simulink model "SoftManipulatorModel"  (R2019a)
settings: Solver=VariableStepAuto  StartTime=0.0  StopTime=100  FixedStep=0.01  RelTol=1e-3
undefined symbols (not defined in the file): d, dq_init, k, l, m, q_init
libraries: dspinverses x1
(part 1 of 2)
settings Model: Creator=Shaon  LastModifiedBy=Shaon

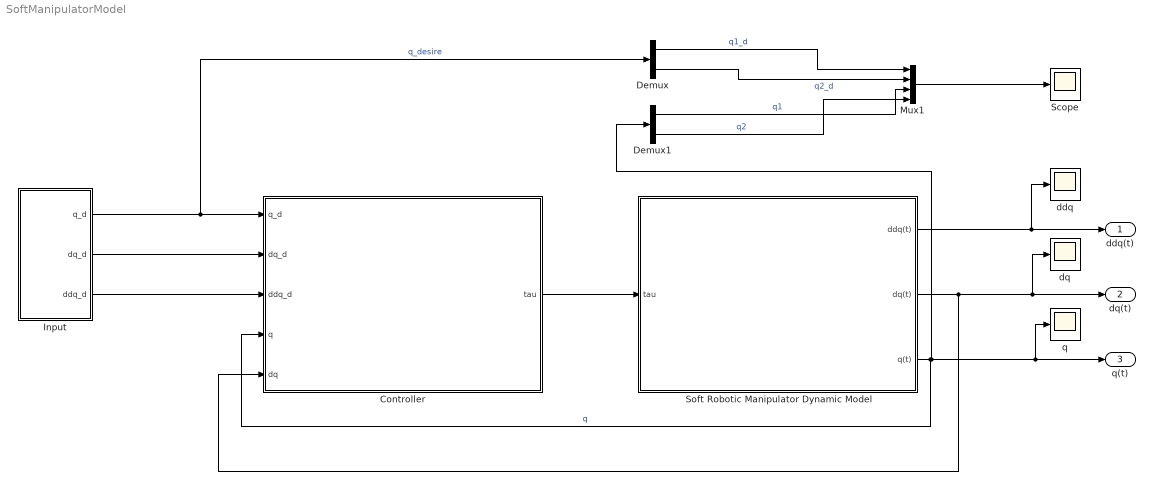
== system SoftManipulatorModel ==
  Controller : Subsystem
  Demux : Demux  Outputs=2
  Demux1 : Demux  Outputs=2
  Input : Subsystem
  Mux1 : Mux
  Scope : Scope
  Soft Robotic Manipulator Dynamic Model : Subsystem
  ddq : Scope
  dq : Scope
  q : Scope
  ddq(t) : Outport
  dq(t) : Outport  Port=2
  q(t) : Outport  Port=3
  wires:
  Soft Robotic Manipulator Dynamic Model/1(ddq(t)) -> ddq/1, ddq(t)/1
  Soft Robotic Manipulator Dynamic Model/2(dq(t)) -> Controller/5(dq), dq/1, dq(t)/1
  Soft Robotic Manipulator Dynamic Model/3(q(t)) -> Demux1/1, q/1, q(t)/1, Controller/4(q)  "q"
  Controller/1(tau) -> Soft Robotic Manipulator Dynamic Model/1(tau)
  Input/1(q_d) -> Demux/1, Controller/1(q_d)  "q_desire"
  Input/2(dq_d) -> Controller/2(dq_d)
  Input/3(ddq_d) -> Controller/3(ddq_d)
  Mux1/1 -> Scope/1
  Demux/1 -> Mux1/1  "q1_d"
  Demux/2 -> Mux1/2  "q2_d"
  Demux1/1 -> Mux1/3  "q1"
  Demux1/2 -> Mux1/4  "q2"

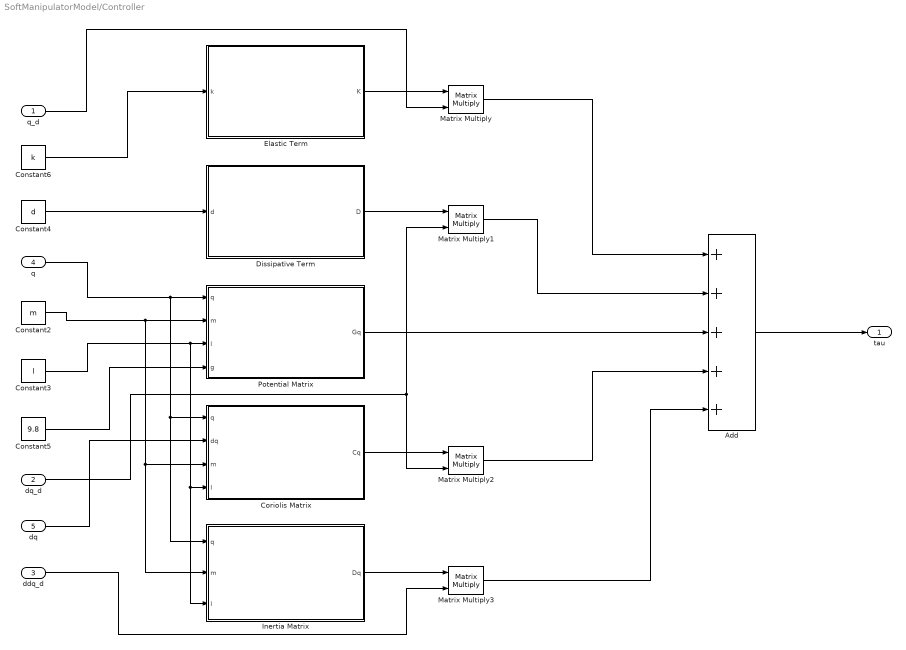
== system SoftManipulatorModel/Controller ==
  q_d : Inport
  dq_d : Inport  Port=2
  ddq_d : Inport  Port=3
  q : Inport  Port=4
  dq : Inport  Port=5
  " Dissipative Term" : MATLAB Function  TreatAsAtomicUnit=on
  Add : Sum  Inputs=+++++
  Constant2 : Constant  Value=m
  Constant3 : Constant  Value=l
  Constant4 : Constant  Value=d
  Constant5 : Constant  Value=9.8
  Constant6 : Constant  Value=k
  Coriolis Matrix : MATLAB Function  TreatAsAtomicUnit=on
  Elastic Term : MATLAB Function  TreatAsAtomicUnit=on
  Inertia Matrix : MATLAB Function  TreatAsAtomicUnit=on
  Matrix Multiply{,1..3} (4 alike) : Product  Multiplication=Matrix(*)
  Potential Matrix : MATLAB Function  TreatAsAtomicUnit=on
  tau : Outport
  wires:
  Elastic Term/1(K) -> Matrix Multiply/1
  " Dissipative Term"/1(D) -> Matrix Multiply1/1
  Potential Matrix/1(Gq) -> Add/3
  Matrix Multiply/1 -> Add/1
  Matrix Multiply1/1 -> Add/2
  Matrix Multiply2/1 -> Add/4
  Matrix Multiply3/1 -> Add/5
  Add/1 -> tau/1
  Coriolis Matrix/1(Cq) -> Matrix Multiply2/1
  Inertia Matrix/1(Dq) -> Matrix Multiply3/1
  Constant6/1 -> Elastic Term/1(k)
  q_d/1 -> Matrix Multiply/2
  Constant4/1 -> " Dissipative Term"/1(d)
  dq_d/1 -> Matrix Multiply1/2, Matrix Multiply2/2
  q/1 -> Inertia Matrix/1(q), Coriolis Matrix/1(q), Potential Matrix/1(q)
  Constant2/1 -> Inertia Matrix/2(m), Coriolis Matrix/3(m), Potential Matrix/2(m)
  Constant3/1 -> Potential Matrix/3(l), Inertia Matrix/3(l), Coriolis Matrix/4(l)
  Constant5/1 -> Potential Matrix/4(g)
  dq/1 -> Coriolis Matrix/2(dq)
  ddq_d/1 -> Matrix Multiply3/2

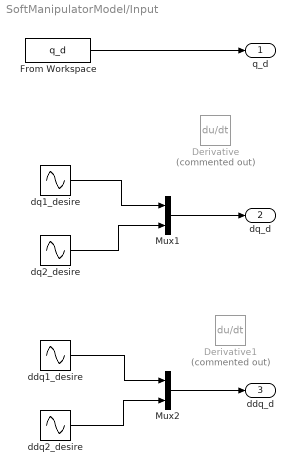
== system SoftManipulatorModel/Input ==
  Derivative : Derivative  Commented=on
  Derivative1 : Derivative  Commented=on
  From Workspace : FromWorkspace  VariableName=q_d  SampleTime=0.1  Interpolate=off  OutputAfterFinalValue=Holding final value
  Mux1 : Mux  Inputs=2
  Mux2 : Mux  Inputs=2
  ddq1_desire : Sin  Amplitude=0  SampleTime=0
  ddq2_desire : Sin  Amplitude=0  SampleTime=0
  dq1_desire : Sin  Amplitude=0  SampleTime=0
  dq2_desire : Sin  Amplitude=0  SampleTime=0
  q_d : Outport
  dq_d : Outport  Port=2
  ddq_d : Outport  Port=3
  wires:
  ddq1_desire/1 -> Mux2/1
  ddq2_desire/1 -> Mux2/2
  Mux2/1 -> ddq_d/1
  Mux1/1 -> dq_d/1
  dq1_desire/1 -> Mux1/1
  dq2_desire/1 -> Mux1/2
  From Workspace/1 -> q_d/1

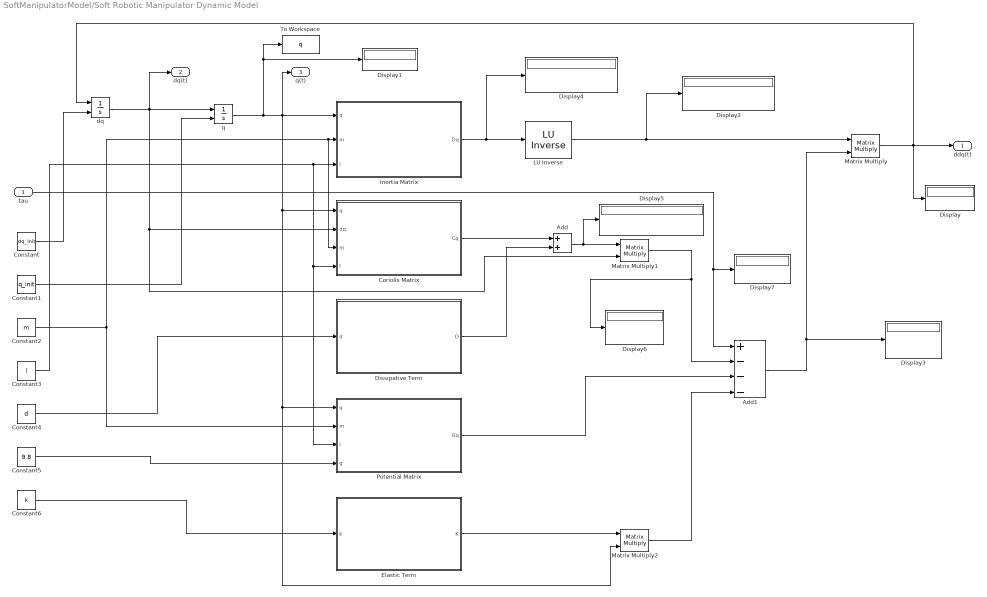
== system SoftManipulatorModel/Soft Robotic Manipulator Dynamic Model ==
  tau : Inport
  " Dissipative Term" : MATLAB Function  TreatAsAtomicUnit=on
  " LU Inverse" : dspinverses/ LU Inverse
      settings: SourceProductName=DSP System Toolbox
  Add : Sum
  Add1 : Sum  Inputs=+---
  Constant : Constant  Value=dq_init
  Constant1 : Constant  Value=q_init
  Constant2 : Constant  Value=m
  Constant3 : Constant  Value=l
  Constant4 : Constant  Value=d
  Constant5 : Constant  Value=9.8
  Constant6 : Constant  Value=k
  Coriolis Matrix : MATLAB Function  TreatAsAtomicUnit=on
  Display{,1..7} (8 alike) : Display
  Elastic Term : MATLAB Function  TreatAsAtomicUnit=on
  Inertia Matrix : MATLAB Function  TreatAsAtomicUnit=on
  Matrix Multiply : Product  Multiplication=Matrix(*)
  Matrix Multiply1 : Product  Multiplication=Matrix(*)
  Matrix Multiply2 : Product  Multiplication=Matrix(*)
  Potential Matrix : MATLAB Function  TreatAsAtomicUnit=on
  To Workspace : ToWorkspace  VariableName=q  SampleTime=-1
      settings: Save2DSignal=2-D array (concatenate along first dimension)
  dq : Integrator  InitialConditionSource=external
  q : Integrator  InitialConditionSource=external
  ddq(t) : Outport
  dq(t) : Outport  Port=2
  q(t) : Outport  Port=3
  wires:
  dq/1 -> dq(t)/1, Coriolis Matrix/2(dq), Matrix Multiply1/2, q/1
  " LU Inverse"/1 -> Display2/1, Matrix Multiply/1
  Coriolis Matrix/1(Cq) -> Add/1
  " Dissipative Term"/1(D) -> Add/2
  Constant5/1 -> Potential Matrix/4(g)
  Constant/1 -> dq/2
  Matrix Multiply1/1 -> Display6/1, Add1/2
  Inertia Matrix/1(Dq) -> Display4/1, " LU Inverse"/1
  tau/1 -> Display7/1, Add1/1
  Potential Matrix/1(Gq) -> Add1/3
  Constant2/1 -> Potential Matrix/2(m), Coriolis Matrix/3(m), Inertia Matrix/2(m)
  Add1/1 -> Matrix Multiply/2, Display3/1
  Constant1/1 -> q/2
  Matrix Multiply/1 -> Display/1, ddq(t)/1, dq/1
  Matrix Multiply2/1 -> Add1/4
  Constant3/1 -> Coriolis Matrix/4(l), Potential Matrix/3(l), Inertia Matrix/3(l)
  Add/1 -> Matrix Multiply1/1, Display5/1
  Constant6/1 -> Elastic Term/1(k)
  Constant4/1 -> " Dissipative Term"/1(d)
  Elastic Term/1(K) -> Matrix Multiply2/1
  q/1 -> Inertia Matrix/1(q), Potential Matrix/1(q), Matrix Multiply2/2, Coriolis Matrix/1(q), q(t)/1, Display1/1, To Workspace/1

== matlab function SoftManipulatorModel/Soft Robotic Manipulator Dynamic Model/Coriolis Matrix ==
  data: q input; Cq output; dq input; m input; l input
function Cq = fcn(q, dq, m, l)

q1 = q(1);
q2 = q(2);
dq1 = dq(1);
dq2 = dq(2);
m1 = m(1);
m2 = m(2);
l1 = l(1);
l2 = l(2);

Cq = zeros(2,2);
% C111 = 0;
% C121 = 0;
% C221 = 0;
% C112 = 0;
% C222 = 0;
% tolerance = 1e-4;
% fake_zero = 1e-3;

% This equation got from Matlab symbolic calculation
% if abs(q1) < tolerance && abs(q2) > tolerance
%     C111 = 0;
%     C121 = -(m2*((l2*sin(conj(q2))*conj(l2)*(cos(q2) - 1))/(4*q2*conj(q2)) - ((l2*cos(q2))/(2*q2) - (l2*sin(q2))/(2*q2^2))*(conj(l1) + (sin(conj(q2))*conj(l2))/(2*conj(q2))) - (l1 + (l2*sin(q2))/(2*q2))*((cos(conj(q2))*conj(l2))/(2*conj(q2)) - (sin(conj(q2))*conj(l2))/(2*conj(q2)^2)) + (l2*conj(l2)*sin(q2)*(cos(conj(q2)) - 1))/(4*q2*conj(q2)) + (l2*conj(l2)*(cos(q2) - 1)*(cos(conj(q2)) - 1))/(4*q2*conj(q2)^2) + (l2*conj(l2)*(cos(q2) - 1)*(cos(conj(q2)) - 1))/(4*q2^2*conj(q2))))/2;
%     C221 = -m2*((l2*sin(q2)*(conj(l1) + (sin(conj(q2))*conj(l2))/(2*conj(q2))))/(2*q2^2) - (l2*cos(q2)*(conj(l1) + (sin(conj(q2))*conj(l2))/(2*conj(q2))))/(2*q2) - (l2*sin(q2)*((cos(conj(q2))*conj(l2))/(2*conj(q2)) - (sin(conj(q2))*conj(l2))/(2*conj(q2)^2)))/(2*q2) + (l2*sin(conj(q2))*conj(l2)*(cos(q2) - 1))/(4*q2*conj(q2)) + (l2*conj(l2)*sin(q2)*(cos(conj(q2)) - 1))/(4*q2*conj(q2)) + (l2*conj(l2)*(cos(q2) - 1)*(cos(conj(q2)) - 1))/(4*q2*conj(q2)^2) + (l2*conj(l2)*(cos(q2) - 1)*(cos(conj(q2)) - 1))/(4*q2^2*conj(q2)));
%     C112 = (m2*((l2*sin(conj(q2))*conj(l2)*(cos(q2) - 1))/(4*q2*conj(q2)) - ((l2*cos(q2))/(2*q2) - (l2*sin(q2))/(2*q2^2))*(conj(l1) + (sin(conj(q2))*conj(l2))/(2*conj(q2))) - (l1 + (l2*sin(q2))/(2*q2))*((cos(conj(q2))*conj(l2))/(2*conj(q2)) - (sin(conj(q2))*conj(l2))/(2*conj(q2)^2)) + (l2*conj(l2)*sin(q2)*(cos(conj(q2)) - 1))/(4*q2*conj(q2)) + (l2*conj(l2)*(cos(q2) - 1)*(cos(conj(q2)) - 1))/(4*q2*conj(q2)^2) + (l2*conj(l2)*(cos(q2) - 1)*(cos(conj(q2)) - 1))/(4*q2^2*conj(q2))))/2;
%     C222 = -(m2*((l2*sin(conj(q2))*conj(l2)*(cos(q2) - 1))/(4*q2*conj(q2)) + (l2*conj(l2)*sin(q2)*(cos(conj(q2)) - 1))/(4*q2*conj(q2)) + (l2*conj(l2)*(cos(q2) - 1)*(cos(conj(q2)) - 1))/(4*q2*conj(q2)^2) + (l2*conj(l2)*(cos(q2) - 1)*(cos(conj(q2)) - 1))/(4*q2^2*conj(q2)) - (l2*cos(conj(q2))*conj(l2)*sin(q2))/(4*q2*conj(q2)) - (l2*sin(conj(q2))*conj(l2)*cos(q2))/(4*q2*conj(q2)) + (l2*sin(conj(q2))*conj(l2)*sin(q2))/(4*q2*conj(q2)^2) + (l2*sin(conj(q2))*conj(l2)*sin(q2))/(4*q2^2*conj(q2))))/2;
% elseif abs(q1) < tolerance && abs(q2) < tolerance
%     C111 = 0;
%     C121 = 0;
%     C221 = 0;
%     C112 = 0;
%     C222 = 0;
% elseif abs(q1) > tolerance && abs(q2) < tolerance
%     C111 = m2*(((sin(conj(q1))*conj(l2))/2 - (conj(l1)*(cos(conj(q1)) - 1))/conj(q1))*((l2*cos(q1))/2 + (l1*sin(q1))/q1 + (l1*(cos(q1) - 1))/q1^2) + ((l2*sin(q1))/2 - (l1*(cos(q1) - 1))/q1)*((cos(conj(q1))*conj(l2))/2 + (sin(conj(q1))*conj(l1))/conj(q1) + (conj(l1)*(cos(conj(q1)) - 1))/conj(q1)^2) - ((cos(conj(q1))*conj(l2))/2 + (sin(conj(q1))*conj(l1))/conj(q1))*((l2*sin(q1))/2 - (l1*cos(q1))/q1 + (l1*sin(q1))/q1^2) - ((l2*cos(q1))/2 + (l1*sin(q1))/q1)*((sin(conj(q1))*conj(l2))/2 - (cos(conj(q1))*conj(l1))/conj(q1) + (sin(conj(q1))*conj(l1))/conj(q1)^2)) - m1*((l1*sin(conj(q1))*conj(l1)*(cos(q1) - 1))/(4*q1*conj(q1)) + (l1*conj(l1)*sin(q1)*(cos(conj(q1)) - 1))/(4*q1*conj(q1)) + (l1*conj(l1)*(cos(q1) - 1)*(cos(conj(q1)) - 1))/(4*q1*conj(q1)^2) + (l1*conj(l1)*(cos(q1) - 1)*(cos(conj(q1)) - 1))/(4*q1^2*conj(q1)) - (l1*cos(conj(q1))*conj(l1)*sin(q1))/(4*q1*conj(q1)) - (l1*sin(conj(q1))*conj(l1)*cos(q1))/(4*q1*conj(q1)) + (l1*sin(conj(q1))*conj(l1)*sin(q1))/(4*q1*conj(q1)^2) + (l1*sin(conj(q1))*conj(l1)*sin(q1))/(4*q1^2*conj(q1)));
%     C121 = 0;
%     C221 = 0;
%     C112 = m2*((cos(conj(q1))*conj(l2)*((l2*sin(q1))/2 - (l1*(cos(q1) - 1))/q1))/2 - (cos(conj(q1))*conj(l2)*((l2*sin(q1))/2 - (l1*cos(q1))/q1 + (l1*sin(q1))/q1^2))/2 + (sin(conj(q1))*conj(l2)*((l2*cos(q1))/2 + (l1*sin(q1))/q1 + (l1*(cos(q1) - 1))/q1^2))/2 - (sin(conj(q1))*conj(l2)*((l2*cos(q1))/2 + (l1*sin(q1))/q1))/2);
%     C222 = 0;
% elseif abs(q1) > tolerance && abs(q2) > tolerance
%     C111 = m2*(((l1*sin(q1))/q1 + (l2*cos(q1)*sin(q2))/(2*q2) + (l2*sin(q1)*(cos(q2) - 1))/(2*q2))*((cos(conj(q1))*conj(l1))/conj(q1) - (sin(conj(q1))*conj(l1))/conj(q1)^2 + (cos(conj(q1))*conj(l2)*(cos(conj(q2)) - 1))/(2*conj(q2)) - (sin(conj(q1))*sin(conj(q2))*conj(l2))/(2*conj(q2))) - ((conj(l1)*(cos(conj(q1)) - 1))/conj(q1) + (cos(conj(q1))*conj(l2)*(cos(conj(q2)) - 1))/(2*conj(q2)) - (sin(conj(q1))*sin(conj(q2))*conj(l2))/(2*conj(q2)))*((l1*sin(q1))/q1 + (l1*(cos(q1) - 1))/q1^2 + (l2*cos(q1)*sin(q2))/(2*q2) + (l2*sin(q1)*(cos(q2) - 1))/(2*q2)) - ((l1*(cos(q1) - 1))/q1 - (l2*sin(q1)*sin(q2))/(2*q2) + (l2*cos(q1)*(cos(q2) - 1))/(2*q2))*((sin(conj(q1))*conj(l1))/conj(q1) + (conj(l1)*(cos(conj(q1)) - 1))/conj(q1)^2 + (sin(conj(q1))*conj(l2)*(cos(conj(q2)) - 1))/(2*conj(q2)) + (cos(conj(q1))*sin(conj(q2))*conj(l2))/(2*conj(q2))) + ((sin(conj(q1))*conj(l1))/conj(q1) + (sin(conj(q1))*conj(l2)*(cos(conj(q2)) - 1))/(2*conj(q2)) + (cos(conj(q1))*sin(conj(q2))*conj(l2))/(2*conj(q2)))*((l1*cos(q1))/q1 - (l1*sin(q1))/q1^2 - (l2*sin(q1)*sin(q2))/(2*q2) + (l2*cos(q1)*(cos(q2) - 1))/(2*q2))) - m1*((l1*sin(conj(q1))*conj(l1)*(cos(q1) - 1))/(4*q1*conj(q1)) + (l1*conj(l1)*sin(q1)*(cos(conj(q1)) - 1))/(4*q1*conj(q1)) + (l1*conj(l1)*(cos(q1) - 1)*(cos(conj(q1)) - 1))/(4*q1*conj(q1)^2) + (l1*conj(l1)*(cos(q1) - 1)*(cos(conj(q1)) - 1))/(4*q1^2*conj(q1)) - (l1*cos(conj(q1))*conj(l1)*sin(q1))/(4*q1*conj(q1)) - (l1*sin(conj(q1))*conj(l1)*cos(q1))/(4*q1*conj(q1)) + (l1*sin(conj(q1))*conj(l1)*sin(q1))/(4*q1*conj(q1)^2) + (l1*sin(conj(q1))*conj(l1)*sin(q1))/(4*q1^2*conj(q1)));
%     C121 = -(m2*(((l1*sin(q1))/q1 + (l2*cos(q1)*sin(q2))/(2*q2) + (l2*sin(q1)*(cos(q2) - 1))/(2*q2))*((sin(conj(q1))*conj(l2)*(cos(conj(q2)) - 1))/(2*conj(q2)^2) - (cos(conj(q1))*cos(conj(q2))*conj(l2))/(2*conj(q2)) + (cos(conj(q1))*sin(conj(q2))*conj(l2))/(2*conj(q2)^2) + (sin(conj(q1))*sin(conj(q2))*conj(l2))/(2*conj(q2))) + ((sin(conj(q1))*conj(l1))/conj(q1) + (sin(conj(q1))*conj(l2)*(cos(conj(q2)) - 1))/(2*conj(q2)) + (cos(conj(q1))*sin(conj(q2))*conj(l2))/(2*conj(q2)))*((l2*cos(q1)*sin(q2))/(2*q2^2) - (l2*cos(q1)*cos(q2))/(2*q2) + (l2*sin(q1)*sin(q2))/(2*q2) + (l2*sin(q1)*(cos(q2) - 1))/(2*q2^2)) + ((l1*(cos(q1) - 1))/q1 - (l2*sin(q1)*sin(q2))/(2*q2) + (l2*cos(q1)*(cos(q2) - 1))/(2*q2))*((cos(conj(q1))*conj(l2)*(cos(conj(q2)) - 1))/(2*conj(q2)^2) + (cos(conj(q1))*sin(conj(q2))*conj(l2))/(2*conj(q2)) + (cos(conj(q2))*sin(conj(q1))*conj(l2))/(2*conj(q2)) - (sin(conj(q1))*sin(conj(q2))*conj(l2))/(2*conj(q2)^2)) + ((conj(l1)*(cos(conj(q1)) - 1))/conj(q1) + (cos(conj(q1))*conj(l2)*(cos(conj(q2)) - 1))/(2*conj(q2)) - (sin(conj(q1))*sin(conj(q2))*conj(l2))/(2*conj(q2)))*((l2*cos(q1)*sin(q2))/(2*q2) + (l2*cos(q2)*sin(q1))/(2*q2) - (l2*sin(q1)*sin(q2))/(2*q2^2) + (l2*cos(q1)*(cos(q2) - 1))/(2*q2^2))))/2;
%     C221 = -m2*(((l2*cos(q1)*sin(q2))/(2*q2) + (l2*sin(q1)*(cos(q2) - 1))/(2*q2))*((sin(conj(q1))*conj(l2)*(cos(conj(q2)) - 1))/(2*conj(q2)^2) - (cos(conj(q1))*cos(conj(q2))*conj(l2))/(2*conj(q2)) + (cos(conj(q1))*sin(conj(q2))*conj(l2))/(2*conj(q2)^2) + (sin(conj(q1))*sin(conj(q2))*conj(l2))/(2*conj(q2))) - ((l2*sin(q1)*sin(q2))/(2*q2) - (l2*cos(q1)*(cos(q2) - 1))/(2*q2))*((cos(conj(q1))*conj(l2)*(cos(conj(q2)) - 1))/(2*conj(q2)^2) + (cos(conj(q1))*sin(conj(q2))*conj(l2))/(2*conj(q2)) + (cos(conj(q2))*sin(conj(q1))*conj(l2))/(2*conj(q2)) - (sin(conj(q1))*sin(conj(q2))*conj(l2))/(2*conj(q2)^2)) + ((sin(conj(q1))*conj(l1))/conj(q1) + (sin(conj(q1))*conj(l2)*(cos(conj(q2)) - 1))/(2*conj(q2)) + (cos(conj(q1))*sin(conj(q2))*conj(l2))/(2*conj(q2)))*((l2*cos(q1)*sin(q2))/(2*q2^2) - (l2*cos(q1)*cos(q2))/(2*q2) + (l2*sin(q1)*sin(q2))/(2*q2) + (l2*sin(q1)*(cos(q2) - 1))/(2*q2^2)) + ((conj(l1)*(cos(conj(q1)) - 1))/conj(q1) + (cos(conj(q1))*conj(l2)*(cos(conj(q2)) - 1))/(2*conj(q2)) - (sin(conj(q1))*sin(conj(q2))*conj(l2))/(2*conj(q2)))*((l2*cos(q1)*sin(q2))/(2*q2) + (l2*cos(q2)*sin(q1))/(2*q2) - (l2*sin(q1)*sin(q2))/(2*q2^2) + (l2*cos(q1)*(cos(q2) - 1))/(2*q2^2)));
%     C112 = (m2*(((l1*sin(q1))/q1 + (l2*cos(q1)*sin(q2))/(2*q2) + (l2*sin(q1)*(cos(q2) - 1))/(2*q2))*((sin(conj(q1))*conj(l2)*(cos(conj(q2)) - 1))/(2*conj(q2)^2) - (cos(conj(q1))*cos(conj(q2))*conj(l2))/(2*conj(q2)) + (cos(conj(q1))*sin(conj(q2))*conj(l2))/(2*conj(q2)^2) + (sin(conj(q1))*sin(conj(q2))*conj(l2))/(2*conj(q2))) + ((sin(conj(q1))*conj(l1))/conj(q1) + (sin(conj(q1))*conj(l2)*(cos(conj(q2)) - 1))/(2*conj(q2)) + (cos(conj(q1))*sin(conj(q2))*conj(l2))/(2*conj(q2)))*((l2*cos(q1)*sin(q2))/(2*q2^2) - (l2*cos(q1)*cos(q2))/(2*q2) + (l2*sin(q1)*sin(q2))/(2*q2) + (l2*sin(q1)*(cos(q2) - 1))/(2*q2^2)) + ((l1*(cos(q1) - 1))/q1 - (l2*sin(q1)*sin(q2))/(2*q2) + (l2*cos(q1)*(cos(q2) - 1))/(2*q2))*((cos(conj(q1))*conj(l2)*(cos(conj(q2)) - 1))/(2*conj(q2)^2) + (cos(conj(q1))*sin(conj(q2))*conj(l2))/(2*conj(q2)) + (cos(conj(q2))*sin(conj(q1))*conj(l2))/(2*conj(q2)) - (sin(conj(q1))*sin(conj(q2))*conj(l2))/(2*conj(q2)^2)) + ((conj(l1)*(cos(conj(q1)) - 1))/conj(q1) + (cos(conj(q1))*conj(l2)*(cos(conj(q2)) - 1))/(2*conj(q2)) - (sin(conj(q1))*sin(conj(q2))*conj(l2))/(2*conj(q2)))*((l2*cos(q1)*sin(q2))/(2*q2) + (l2*cos(q2)*sin(q1))/(2*q2) - (l2*sin(q1)*sin(q2))/(2*q2^2) + (l2*cos(q1)*(cos(q2) - 1))/(2*q2^2))))/2 - m2*(((sin(conj(q1))*conj(l2)*(cos(conj(q2)) - 1))/(2*conj(q2)) + (cos(conj(q1))*sin(conj(q2))*conj(l2))/(2*conj(q2)))*((l1*(cos(q1) - 1))/q1 - (l2*sin(q1)*sin(q2))/(2*q2) + (l2*cos(q1)*(cos(q2) - 1))/(2*q2)) - ((sin(conj(q1))*conj(l2)*(cos(conj(q2)) - 1))/(2*conj(q2)) + (cos(conj(q1))*sin(conj(q2))*conj(l2))/(2*conj(q2)))*((l1*cos(q1))/q1 - (l1*sin(q1))/q1^2 - (l2*sin(q1)*sin(q2))/(2*q2) + (l2*cos(q1)*(cos(q2) - 1))/(2*q2)) + ((cos(conj(q1))*conj(l2)*(cos(conj(q2)) - 1))/(2*conj(q2)) - (sin(conj(q1))*sin(conj(q2))*conj(l2))/(2*conj(q2)))*((l1*sin(q1))/q1 + (l1*(cos(q1) - 1))/q1^2 + (l2*cos(q1)*sin(q2))/(2*q2) + (l2*sin(q1)*(cos(q2) - 1))/(2*q2)) - ((cos(conj(q1))*conj(l2)*(cos(conj(q2)) - 1))/(2*conj(q2)) - (sin(conj(q1))*sin(conj(q2))*conj(l2))/(2*conj(q2)))*((l1*sin(q1))/q1 + (l2*cos(q1)*sin(q2))/(2*q2) + (l2*sin(q1)*(cos(q2) - 1))/(2*q2)));
%     C222 = -(m2*(((l2*cos(q1)*sin(q2))/(2*q2) + (l2*sin(q1)*(cos(q2) - 1))/(2*q2))*((sin(conj(q1))*conj(l2)*(cos(conj(q2)) - 1))/(2*conj(q2)^2) - (cos(conj(q1))*cos(conj(q2))*conj(l2))/(2*conj(q2)) + (cos(conj(q1))*sin(conj(q2))*conj(l2))/(2*conj(q2)^2) + (sin(conj(q1))*sin(conj(q2))*conj(l2))/(2*conj(q2))) - ((l2*sin(q1)*sin(q2))/(2*q2) - (l2*cos(q1)*(cos(q2) - 1))/(2*q2))*((cos(conj(q1))*conj(l2)*(cos(conj(q2)) - 1))/(2*conj(q2)^2) + (cos(conj(q1))*sin(conj(q2))*conj(l2))/(2*conj(q2)) + (cos(conj(q2))*sin(conj(q1))*conj(l2))/(2*conj(q2)) - (sin(conj(q1))*sin(conj(q2))*conj(l2))/(2*conj(q2)^2)) + ((cos(conj(q1))*conj(l2)*(cos(conj(q2)) - 1))/(2*conj(q2)) - (sin(conj(q1))*sin(conj(q2))*conj(l2))/(2*conj(q2)))*((l2*cos(q1)*sin(q2))/(2*q2) + (l2*cos(q2)*sin(q1))/(2*q2) - (l2*sin(q1)*sin(q2))/(2*q2^2) + (l2*cos(q1)*(cos(q2) - 1))/(2*q2^2)) + ((sin(conj(q1))*conj(l2)*(cos(conj(q2)) - 1))/(2*conj(q2)) + (cos(conj(q1))*sin(conj(q2))*conj(l2))/(2*conj(q2)))*((l2*cos(q1)*sin(q2))/(2*q2^2) - (l2*cos(q1)*cos(q2))/(2*q2) + (l2*sin(q1)*sin(q2))/(2*q2) + (l2*sin(q1)*(cos(q2) - 1))/(2*q2^2))))/2;
% end

% if abs(q1) < tolerance && abs(q2) > tolerance
%     if q1 < 0
%         q1 = -fake_zero;
%     else
%         q1 = fake_zero;
%     end
% elseif abs(q1) < tolerance && abs(q2) < tolerance
%     if q1 < 0
%         q1 = -fake_zero;
%     else
%         q1 = fake_zero;
%     end
%     
%     if q2 < 0
%         q2 = -fake_zero;
%     else
%         q2 = fake_zero;
%     end
% elseif abs(q1) > tolerance && abs(q2) < tolerance
%     if q2 < 0
%         q2 = -fake_zero;
%     else
%         q2 = fake_zero;
%     end
% end

C111 = m2*(((l1*sin(q1))/q1 + (l2*cos(q1)*sin(q2))/(2*q2) + (l2*sin(q1)*(cos(q2) - 1))/(2*q2))*((cos(conj(q1))*conj(l1))/conj(q1) - (sin(conj(q1))*conj(l1))/conj(q1)^2 + (cos(conj(q1))*conj(l2)*(cos(conj(q2)) - 1))/(2*conj(q2)) - (sin(conj(q1))*sin(conj(q2))*conj(l2))/(2*conj(q2))) - ((conj(l1)*(cos(conj(q1)) - 1))/conj(q1) + (cos(conj(q1))*conj(l2)*(cos(conj(q2)) - 1))/(2*conj(q2)) - (sin(conj(q1))*sin(conj(q2))*conj(l2))/(2*conj(q2)))*((l1*sin(q1))/q1 + (l1*(cos(q1) - 1))/q1^2 + (l2*cos(q1)*sin(q2))/(2*q2) + (l2*sin(q1)*(cos(q2) - 1))/(2*q2)) - ((l1*(cos(q1) - 1))/q1 - (l2*sin(q1)*sin(q2))/(2*q2) + (l2*cos(q1)*(cos(q2) - 1))/(2*q2))*((sin(conj(q1))*conj(l1))/conj(q1) + (conj(l1)*(cos(conj(q1)) - 1))/conj(q1)^2 + (sin(conj(q1))*conj(l2)*(cos(conj(q2)) - 1))/(2*conj(q2)) + (cos(conj(q1))*sin(conj(q2))*conj(l2))/(2*conj(q2))) + ((sin(conj(q1))*conj(l1))/conj(q1) + (sin(conj(q1))*conj(l2)*(cos(conj(q2)) - 1))/(2*conj(q2)) + (cos(conj(q1))*sin(conj(q2))*conj(l2))/(2*conj(q2)))*((l1*cos(q1))/q1 - (l1*sin(q1))/q1^2 - (l2*sin(q1)*sin(q2))/(2*q2) + (l2*cos(q1)*(cos(q2) - 1))/(2*q2))) - m1*((l1*sin(conj(q1))*conj(l1)*(cos(q1) - 1))/(4*q1*conj(q1)) + (l1*conj(l1)*sin(q1)*(cos(conj(q1)) - 1))/(4*q1*conj(q1)) + (l1*conj(l1)*(cos(q1) - 1)*(cos(conj(q1)) - 1))/(4*q1*conj(q1)^2) + (l1*conj(l1)*(cos(q1) - 1)*(cos(conj(q1)) - 1))/(4*q1^2*conj(q1)) - (l1*cos(conj(q1))*conj(l1)*sin(q1))/(4*q1*conj(q1)) - (l1*sin(conj(q1))*conj(l1)*cos(q1))/(4*q1*conj(q1)) + (l1*sin(conj(q1))*conj(l1)*sin(q1))/(4*q1*conj(q1)^2) + (l1*sin(conj(q1))*conj(l1)*sin(q1))/(4*q1^2*conj(q1)));
C121 = -(m2*(((l1*sin(q1))/q1 + (l2*cos(q1)*sin(q2))/(2*q2) + (l2*sin(q1)*(cos(q2) - 1))/(2*q2))*((sin(conj(q1))*conj(l2)*(cos(conj(q2)) - 1))/(2*conj(q2)^2) - (cos(conj(q1))*cos(conj(q2))*conj(l2))/(2*conj(q2)) + (cos(conj(q1))*sin(conj(q2))*conj(l2))/(2*conj(q2)^2) + (sin(conj(q1))*sin(conj(q2))*conj(l2))/(2*conj(q2))) + ((sin(conj(q1))*conj(l1))/conj(q1) + (sin(conj(q1))*conj(l2)*(cos(conj(q2)) - 1))/(2*conj(q2)) + (cos(conj(q1))*sin(conj(q2))*conj(l2))/(2*conj(q2)))*((l2*cos(q1)*sin(q2))/(2*q2^2) - (l2*cos(q1)*cos(q2))/(2*q2) + (l2*sin(q1)*sin(q2))/(2*q2) + (l2*sin(q1)*(cos(q2) - 1))/(2*q2^2)) + ((l1*(cos(q1) - 1))/q1 - (l2*sin(q1)*sin(q2))/(2*q2) + (l2*cos(q1)*(cos(q2) - 1))/(2*q2))*((cos(conj(q1))*conj(l2)*(cos(conj(q2)) - 1))/(2*conj(q2)^2) + (cos(conj(q1))*sin(conj(q2))*conj(l2))/(2*conj(q2)) + (cos(conj(q2))*sin(conj(q1))*conj(l2))/(2*conj(q2)) - (sin(conj(q1))*sin(conj(q2))*conj(l2))/(2*conj(q2)^2)) + ((conj(l1)*(cos(conj(q1)) - 1))/conj(q1) + (cos(conj(q1))*conj(l2)*(cos(conj(q2)) - 1))/(2*conj(q2)) - (sin(conj(q1))*sin(conj(q2))*conj(l2))/(2*conj(q2)))*((l2*cos(q1)*sin(q2))/(2*q2) + (l2*cos(q2)*sin(q1))/(2*q2) - (l2*sin(q1)*sin(q2))/(2*q2^2) + (l2*cos(q1)*(cos(q2) - 1))/(2*q2^2))))/2;
C221 = -m2*(((l2*cos(q1)*sin(q2))/(2*q2) + (l2*sin(q1)*(cos(q2) - 1))/(2*q2))*((sin(conj(q1))*conj(l2)*(cos(conj(q2)) - 1))/(2*conj(q2)^2) - (cos(conj(q1))*cos(conj(q2))*conj(l2))/(2*conj(q2)) + (cos(conj(q1))*sin(conj(q2))*conj(l2))/(2*conj(q2)^2) + (sin(conj(q1))*sin(conj(q2))*conj(l2))/(2*conj(q2))) - ((l2*sin(q1)*sin(q2))/(2*q2) - (l2*cos(q1)*(cos(q2) - 1))/(2*q2))*((cos(conj(q1))*conj(l2)*(cos(conj(q2)) - 1))/(2*conj(q2)^2) + (cos(conj(q1))*sin(conj(q2))*conj(l2))/(2*conj(q2)) + (cos(conj(q2))*sin(conj(q1))*conj(l2))/(2*conj(q2)) - (sin(conj(q1))*sin(conj(q2))*conj(l2))/(2*conj(q2)^2)) + ((sin(conj(q1))*conj(l1))/conj(q1) + (sin(conj(q1))*conj(l2)*(cos(conj(q2)) - 1))/(2*conj(q2)) + (cos(conj(q1))*sin(conj(q2))*conj(l2))/(2*conj(q2)))*((l2*cos(q1)*sin(q2))/(2*q2^2) - (l2*cos(q1)*cos(q2))/(2*q2) + (l2*sin(q1)*sin(q2))/(2*q2) + (l2*sin(q1)*(cos(q2) - 1))/(2*q2^2)) + ((conj(l1)*(cos(conj(q1)) - 1))/conj(q1) + (cos(conj(q1))*conj(l2)*(cos(conj(q2)) - 1))/(2*conj(q2)) - (sin(conj(q1))*sin(conj(q2))*conj(l2))/(2*conj(q2)))*((l2*cos(q1)*sin(q2))/(2*q2) + (l2*cos(q2)*sin(q1))/(2*q2) - (l2*sin(q1)*sin(q2))/(2*q2^2) + (l2*cos(q1)*(cos(q2) - 1))/(2*q2^2)));
C112 = (m2*(((l1*sin(q1))/q1 + (l2*cos(q1)*sin(q2))/(2*q2) + (l2*sin(q1)*(cos(q2) - 1))/(2*q2))*((sin(conj(q1))*conj(l2)*(cos(conj(q2)) - 1))/(2*conj(q2)^2) - (cos(conj(q1))*cos(conj(q2))*conj(l2))/(2*conj(q2)) + (cos(conj(q1))*sin(conj(q2))*conj(l2))/(2*conj(q2)^2) + (sin(conj(q1))*sin(conj(q2))*conj(l2))/(2*conj(q2))) + ((sin(conj(q1))*conj(l1))/conj(q1) + (sin(conj(q1))*conj(l2)*(cos(conj(q2)) - 1))/(2*conj(q2)) + (cos(conj(q1))*sin(conj(q2))*conj(l2))/(2*conj(q2)))*((l2*cos(q1)*sin(q2))/(2*q2^2) - (l2*cos(q1)*cos(q2))/(2*q2) + (l2*sin(q1)*sin(q2))/(2*q2) + (l2*sin(q1)*(cos(q2) - 1))/(2*q2^2)) + ((l1*(cos(q1) - 1))/q1 - (l2*sin(q1)*sin(q2))/(2*q2) + (l2*cos(q1)*(cos(q2) - 1))/(2*q2))*((cos(conj(q1))*conj(l2)*(cos(conj(q2)) - 1))/(2*conj(q2)^2) + (cos(conj(q1))*sin(conj(q2))*conj(l2))/(2*conj(q2)) + (cos(conj(q2))*sin(conj(q1))*conj(l2))/(2*conj(q2)) - (sin(conj(q1))*sin(conj(q2))*conj(l2))/(2*conj(q2)^2)) + ((conj(l1)*(cos(conj(q1)) - 1))/conj(q1) + (cos(conj(q1))*conj(l2)*(cos(conj(q2)) - 1))/(2*conj(q2)) - (sin(conj(q1))*sin(conj(q2))*conj(l2))/(2*conj(q2)))*((l2*cos(q1)*sin(q2))/(2*q2) + (l2*cos(q2)*sin(q1))/(2*q2) - (l2*sin(q1)*sin(q2))/(2*q2^2) + (l2*cos(q1)*(cos(q2) - 1))/(2*q2^2))))/2 - m2*(((sin(conj(q1))*conj(l2)*(cos(conj(q2)) - 1))/(2*conj(q2)) + (cos(conj(q1))*sin(conj(q2))*conj(l2))/(2*conj(q2)))*((l1*(cos(q1) - 1))/q1 - (l2*sin(q1)*sin(q2))/(2*q2) + (l2*cos(q1)*(cos(q2) - 1))/(2*q2)) - ((sin(conj(q1))*conj(l2)*(cos(conj(q2)) - 1))/(2*conj(q2)) + (cos(conj(q1))*sin(conj(q2))*conj(l2))/(2*conj(q2)))*((l1*cos(q1))/q1 - (l1*sin(q1))/q1^2 - (l2*sin(q1)*sin(q2))/(2*q2) + (l2*cos(q1)*(cos(q2) - 1))/(2*q2)) + ((cos(conj(q1))*conj(l2)*(cos(conj(q2)) - 1))/(2*conj(q2)) - (sin(conj(q1))*sin(conj(q2))*conj(l2))/(2*conj(q2)))*((l1*sin(q1))/q1 + (l1*(cos(q1) - 1))/q1^2 + (l2*cos(q1)*sin(q2))/(2*q2) + (l2*sin(q1)*(cos(q2) - 1))/(2*q2)) - ((cos(conj(q1))*conj(l2)*(cos(conj(q2)) - 1))/(2*conj(q2)) - (sin(conj(q1))*sin(conj(q2))*conj(l2))/(2*conj(q2)))*((l1*sin(q1))/q1 + (l2*cos(q1)*sin(q2))/(2*q2) + (l2*sin(q1)*(cos(q2) - 1))/(2*q2)));
C222 = -(m2*(((l2*cos(q1)*sin(q2))/(2*q2) + (l2*sin(q1)*(cos(q2) - 1))/(2*q2))*((sin(conj(q1))*conj(l2)*(cos(conj(q2)) - 1))/(2*conj(q2)^2) - (cos(conj(q1))*cos(conj(q2))*conj(l2))/(2*conj(q2)) + (cos(conj(q1))*sin(conj(q2))*conj(l2))/(2*conj(q2)^2) + (sin(conj(q1))*sin(conj(q2))*conj(l2))/(2*conj(q2))) - ((l2*sin(q1)*sin(q2))/(2*q2) - (l2*cos(q1)*(cos(q2) - 1))/(2*q2))*((cos(conj(q1))*conj(l2)*(cos(conj(q2)) - 1))/(2*conj(q2)^2) + (cos(conj(q1))*sin(conj(q2))*conj(l2))/(2*conj(q2)) + (cos(conj(q2))*sin(conj(q1))*conj(l2))/(2*conj(q2)) - (sin(conj(q1))*sin(conj(q2))*conj(l2))/(2*conj(q2)^2)) + ((cos(conj(q1))*conj(l2)*(cos(conj(q2)) - 1))/(2*conj(q2)) - (sin(conj(q1))*sin(conj(q2))*conj(l2))/(2*conj(q2)))*((l2*cos(q1)*sin(q2))/(2*q2) + (l2*cos(q2)*sin(q1))/(2*q2) - (l2*sin(q1)*sin(q2))/(2*q2^2) + (l2*cos(q1)*(cos(q2) - 1))/(2*q2^2)) + ((sin(conj(q1))*conj(l2)*(cos(conj(q2)) - 1))/(2*conj(q2)) + (cos(conj(q1))*sin(conj(q2))*conj(l2))/(2*conj(q2)))*((l2*cos(q1)*sin(q2))/(2*q2^2) - (l2*cos(q1)*cos(q2))/(2*q2) + (l2*sin(q1)*sin(q2))/(2*q2) + (l2*sin(q1)*(cos(q2) - 1))/(2*q2^2))))/2;

Cq(1,1) = C111 * dq1;
Cq(1,2) = 2 * C121 * dq1 + C221 * dq2;
Cq(2,1) = C112 * dq1;
Cq(2,2) = C222 * dq2;

% for i = 1:2
%     for j = 1:2
%         if Cq(i,j) < tolerance
%             Cq(i,j) = 0;
%         end
%     end
% end

== matlab function SoftManipulatorModel/Soft Robotic Manipulator Dynamic Model/Inertia Matrix ==
  data: q input; Dq output; m input; l input
function Dq = fcn(q,m,l)

q1 = q(1);
q2 = q(2);
m1 = m(1);
m2 = m(2);
l1 = l(1);
l2 = l(2);

Dq = zeros(2,2);
% fake_zero = 1e-3;
% tolerance = 1e-6;

% This equation got from Matlab symbolic calculation
% if abs(q1) < tolerance && abs(q2) > tolerance
%     Dq(1,1) = m2*((l1 + (l2*sin(q2))/(2*q2))*(conj(l1) + (sin(conj(q2))*conj(l2))/(2*conj(q2))) + (l2*conj(l2)*(cos(q2) - 1)*(cos(conj(q2)) - 1))/(4*q2*conj(q2))) + (l1*m1*conj(l1))/4;
%     Dq(1,2) = m2*((l2*sin(q2)*(conj(l1) + (sin(conj(q2))*conj(l2))/(2*conj(q2))))/(2*q2) + (l2*conj(l2)*(cos(q2) - 1)*(cos(conj(q2)) - 1))/(4*q2*conj(q2)));
%     Dq(2,1) = m2*((sin(conj(q2))*conj(l2)*(l1 + (l2*sin(q2))/(2*q2)))/(2*conj(q2)) + (l2*conj(l2)*(cos(q2) - 1)*(cos(conj(q2)) - 1))/(4*q2*conj(q2)));
%     Dq(2,2) = m2*((l2*conj(l2)*(cos(q2) - 1)*(cos(conj(q2)) - 1))/(4*q2*conj(q2)) + (l2*sin(conj(q2))*conj(l2)*sin(q2))/(4*q2*conj(q2)));
% elseif abs(q1) < tolerance && abs(q2) < tolerance
%     Dq(1,1) = (l1*m1*conj(l1))/4 + m2*(conj(l1) + conj(l2)/2)*(l1 + l2/2);
%     Dq(1,2) = (l2*m2*(conj(l1) + conj(l2)/2))/2;
%     Dq(2,1) = (m2*conj(l2)*(l1 + l2/2))/2;
%     Dq(2,2) = (l2*m2*conj(l2))/4;
% elseif abs(q1) > tolerance && abs(q2) < tolerance
%     Dq(1,1) = m1*((l1*conj(l1)*(cos(q1) - 1)*(cos(conj(q1)) - 1))/(4*q1*conj(q1)) + (l1*sin(conj(q1))*conj(l1)*sin(q1))/(4*q1*conj(q1))) + m2*(((sin(conj(q1))*conj(l2))/2 - (conj(l1)*(cos(conj(q1)) - 1))/conj(q1))*((l2*sin(q1))/2 - (l1*(cos(q1) - 1))/q1) + ((cos(conj(q1))*conj(l2))/2 + (sin(conj(q1))*conj(l1))/conj(q1))*((l2*cos(q1))/2 + (l1*sin(q1))/q1));
%     Dq(1,2) = m2*((l2*cos(q1)*((cos(conj(q1))*conj(l2))/2 + (sin(conj(q1))*conj(l1))/conj(q1)))/2 + (l2*sin(q1)*((sin(conj(q1))*conj(l2))/2 - (conj(l1)*(cos(conj(q1)) - 1))/conj(q1)))/2);
%     Dq(2,1) = m2*((sin(conj(q1))*conj(l2)*((l2*sin(q1))/2 - (l1*(cos(q1) - 1))/q1))/2 + (cos(conj(q1))*conj(l2)*((l2*cos(q1))/2 + (l1*sin(q1))/q1))/2);
%     Dq(2,2) = m2*((l2*cos(conj(q1))*conj(l2)*cos(q1))/4 + (l2*sin(conj(q1))*conj(l2)*sin(q1))/4);
% elseif abs(q1) > tolerance && abs(q2) > tolerance
%     Dq(1,1) = m2*(((conj(l1)*(cos(conj(q1)) - 1))/conj(q1) + (cos(conj(q1))*conj(l2)*(cos(conj(q2)) - 1))/(2*conj(q2)) - (sin(conj(q1))*sin(conj(q2))*conj(l2))/(2*conj(q2)))*((l1*(cos(q1) - 1))/q1 - (l2*sin(q1)*sin(q2))/(2*q2) + (l2*cos(q1)*(cos(q2) - 1))/(2*q2)) + ((l1*sin(q1))/q1 + (l2*cos(q1)*sin(q2))/(2*q2) + (l2*sin(q1)*(cos(q2) - 1))/(2*q2))*((sin(conj(q1))*conj(l1))/conj(q1) + (sin(conj(q1))*conj(l2)*(cos(conj(q2)) - 1))/(2*conj(q2)) + (cos(conj(q1))*sin(conj(q2))*conj(l2))/(2*conj(q2)))) + m1*((l1*conj(l1)*(cos(q1) - 1)*(cos(conj(q1)) - 1))/(4*q1*conj(q1)) + (l1*sin(conj(q1))*conj(l1)*sin(q1))/(4*q1*conj(q1)));
%     Dq(1,2) = m2*(((l2*cos(q1)*sin(q2))/(2*q2) + (l2*sin(q1)*(cos(q2) - 1))/(2*q2))*((sin(conj(q1))*conj(l1))/conj(q1) + (sin(conj(q1))*conj(l2)*(cos(conj(q2)) - 1))/(2*conj(q2)) + (cos(conj(q1))*sin(conj(q2))*conj(l2))/(2*conj(q2))) - ((l2*sin(q1)*sin(q2))/(2*q2) - (l2*cos(q1)*(cos(q2) - 1))/(2*q2))*((conj(l1)*(cos(conj(q1)) - 1))/conj(q1) + (cos(conj(q1))*conj(l2)*(cos(conj(q2)) - 1))/(2*conj(q2)) - (sin(conj(q1))*sin(conj(q2))*conj(l2))/(2*conj(q2))));
%     Dq(2,1) = m2*(((sin(conj(q1))*conj(l2)*(cos(conj(q2)) - 1))/(2*conj(q2)) + (cos(conj(q1))*sin(conj(q2))*conj(l2))/(2*conj(q2)))*((l1*sin(q1))/q1 + (l2*cos(q1)*sin(q2))/(2*q2) + (l2*sin(q1)*(cos(q2) - 1))/(2*q2)) + ((cos(conj(q1))*conj(l2)*(cos(conj(q2)) - 1))/(2*conj(q2)) - (sin(conj(q1))*sin(conj(q2))*conj(l2))/(2*conj(q2)))*((l1*(cos(q1) - 1))/q1 - (l2*sin(q1)*sin(q2))/(2*q2) + (l2*cos(q1)*(cos(q2) - 1))/(2*q2)));
%     Dq(2,2) = m2*(((l2*cos(q1)*sin(q2))/(2*q2) + (l2*sin(q1)*(cos(q2) - 1))/(2*q2))*((sin(conj(q1))*conj(l2)*(cos(conj(q2)) - 1))/(2*conj(q2)) + (cos(conj(q1))*sin(conj(q2))*conj(l2))/(2*conj(q2))) - ((l2*sin(q1)*sin(q2))/(2*q2) - (l2*cos(q1)*(cos(q2) - 1))/(2*q2))*((cos(conj(q1))*conj(l2)*(cos(conj(q2)) - 1))/(2*conj(q2)) - (sin(conj(q1))*sin(conj(q2))*conj(l2))/(2*conj(q2))));
% end

% if abs(q1) < tolerance && abs(q2) > tolerance
%     if q1 < 0
%         q1 = -fake_zero;
%     else
%         q1 = fake_zero;
%     end
% elseif abs(q1) < tolerance && abs(q2) < tolerance
%     if q1 < 0
%         q1 = -fake_zero;
%     else
%         q1 = fake_zero;
%     end
%     
%     if q2 < 0
%         q2 = -fake_zero;
%     else
%         q2 = fake_zero;
%     end
% elseif abs(q1) > tolerance && abs(q2) < tolerance
%     if q2 < 0
%         q2 = -fake_zero;
%     else
%         q2 = fake_zero;
%     end
% end

Dq(1,1) = m2*(((conj(l1)*(cos(conj(q1)) - 1))/conj(q1) + (cos(conj(q1))*conj(l2)*(cos(conj(q2)) - 1))/(2*conj(q2)) - (sin(conj(q1))*sin(conj(q2))*conj(l2))/(2*conj(q2)))*((l1*(cos(q1) - 1))/q1 - (l2*sin(q1)*sin(q2))/(2*q2) + (l2*cos(q1)*(cos(q2) - 1))/(2*q2)) + ((l1*sin(q1))/q1 + (l2*cos(q1)*sin(q2))/(2*q2) + (l2*sin(q1)*(cos(q2) - 1))/(2*q2))*((sin(conj(q1))*conj(l1))/conj(q1) + (sin(conj(q1))*conj(l2)*(cos(conj(q2)) - 1))/(2*conj(q2)) + (cos(conj(q1))*sin(conj(q2))*conj(l2))/(2*conj(q2)))) + m1*((l1*conj(l1)*(cos(q1) - 1)*(cos(conj(q1)) - 1))/(4*q1*conj(q1)) + (l1*sin(conj(q1))*conj(l1)*sin(q1))/(4*q1*conj(q1)));
Dq(1,2) = m2*(((l2*cos(q1)*sin(q2))/(2*q2) + (l2*sin(q1)*(cos(q2) - 1))/(2*q2))*((sin(conj(q1))*conj(l1))/conj(q1) + (sin(conj(q1))*conj(l2)*(cos(conj(q2)) - 1))/(2*conj(q2)) + (cos(conj(q1))*sin(conj(q2))*conj(l2))/(2*conj(q2))) - ((l2*sin(q1)*sin(q2))/(2*q2) - (l2*cos(q1)*(cos(q2) - 1))/(2*q2))*((conj(l1)*(cos(conj(q1)) - 1))/conj(q1) + (cos(conj(q1))*conj(l2)*(cos(conj(q2)) - 1))/(2*conj(q2)) - (sin(conj(q1))*sin(conj(q2))*conj(l2))/(2*conj(q2))));
Dq(2,1) = m2*(((sin(conj(q1))*conj(l2)*(cos(conj(q2)) - 1))/(2*conj(q2)) + (cos(conj(q1))*sin(conj(q2))*conj(l2))/(2*conj(q2)))*((l1*sin(q1))/q1 + (l2*cos(q1)*sin(q2))/(2*q2) + (l2*sin(q1)*(cos(q2) - 1))/(2*q2)) + ((cos(conj(q1))*conj(l2)*(cos(conj(q2)) - 1))/(2*conj(q2)) - (sin(conj(q1))*sin(conj(q2))*conj(l2))/(2*conj(q2)))*((l1*(cos(q1) - 1))/q1 - (l2*sin(q1)*sin(q2))/(2*q2) + (l2*cos(q1)*(cos(q2) - 1))/(2*q2)));
Dq(2,2) = m2*(((l2*cos(q1)*sin(q2))/(2*q2) + (l2*sin(q1)*(cos(q2) - 1))/(2*q2))*((sin(conj(q1))*conj(l2)*(cos(conj(q2)) - 1))/(2*conj(q2)) + (cos(conj(q1))*sin(conj(q2))*conj(l2))/(2*conj(q2))) - ((l2*sin(q1)*sin(q2))/(2*q2) - (l2*cos(q1)*(cos(q2) - 1))/(2*q2))*((cos(conj(q1))*conj(l2)*(cos(conj(q2)) - 1))/(2*conj(q2)) - (sin(conj(q1))*sin(conj(q2))*conj(l2))/(2*conj(q2))));

% for i = 1:2
%     for j = 1:2
%         if Dq(i,j) < tolerance
%             Dq(i,j) = fake_zero;
%         end
%     end
% end

== matlab function SoftManipulatorModel/Soft Robotic Manipulator Dynamic Model/Potential Matrix ==
  data: q input; Gq output; m input; l input; g input
function Gq = fcn(q, m, l, g)

q1 = q(1);
q2 = q(2);
m1 = m(1);
m2 = m(2);
l1 = l(1);
l2 = l(2);

Gq = zeros(2,1);
% tolerance = 1e-4;
% fake_zero = 1e-3;

% This equation got from Matlab symbolic calculation
% if abs(q1) < tolerance && abs(q2) > tolerance
%     Gq(1,1) = 0;
%     Gq(2,1) = (g*l2*m2*sin(q2))/(2*q2) + (g*l2*m2*(cos(q2) - 1))/(2*q2^2);
% elseif abs(q1) < tolerance && abs(q2) < tolerance
%     Gq(1,1) = 0;
%     Gq(2,1) = 0;
% elseif abs(q1) > tolerance && abs(q2) < tolerance
%     Gq(1,1) = g*m2*((l2*cos(q1))/2 + (l1*sin(q1))/q1 + (l1*(cos(q1) - 1))/q1^2) + (g*l1*m1*sin(q1))/(2*q1) + (g*l1*m1*(cos(q1) - 1))/(2*q1^2);
%     Gq(2,1) = 0;
% elseif abs(q1) > tolerance && abs(q2) > tolerance
%     Gq(1,1) = (l1*sin(q1))/q1 + (l1*(cos(q1) - 1))/q1^2 + (l2*sin(q1)*(cos(q2) - 1))/(2*q2) + (g*l1*m1*sin(q1))/(2*q1) + (g*l1*m1*(cos(q1) - 1))/(2*q1^2) + (g*l2*m2*cos(q1)*sin(q2))/(2*q2);
%     Gq(2,1) = (l2*cos(q1)*sin(q2))/(2*q2) + (l2*cos(q1)*(cos(q2) - 1))/(2*q2^2) + (g*l2*m2*cos(q2)*sin(q1))/(2*q2) - (g*l2*m2*sin(q1)*sin(q2))/(2*q2^2);
% end

% if abs(q1) < tolerance && abs(q2) > tolerance
%     if q1 < 0
%         q1 = -fake_zero;
%     else
%         q1 = fake_zero;
%     end
% elseif abs(q1) < tolerance && abs(q2) < tolerance
%     if q1 < 0
%         q1 = -fake_zero;
%     else
%         q1 = fake_zero;
%     end
%     
%     if q2 < 0
%         q2 = -fake_zero;
%     else
%         q2 = fake_zero;
%     end
% elseif abs(q1) > tolerance && abs(q2) < tolerance
%     if q2 < 0
%         q2 = -fake_zero;
%     else
%         q2 = fake_zero;
%     end
% end

% Gq(1,1) = (l1*sin(q1))/q1 + (l1*(cos(q1) - 1))/q1^2 + (l2*sin(q1)*(cos(q2) - 1))/(2*q2) + (g*l1*m1*sin(q1))/(2*q1) + (g*l1*m1*(cos(q1) - 1))/(2*q1^2) + (g*l2*m2*cos(q1)*sin(q2))/(2*q2);
% Gq(2,1) = (l2*cos(q1)*sin(q2))/(2*q2) + (l2*cos(q1)*(cos(q2) - 1))/(2*q2^2) + (g*l2*m2*cos(q2)*sin(q1))/(2*q2) - (g*l2*m2*sin(q1)*sin(q2))/(2*q2^2);

Gq = [0; 0];

== matlab function SoftManipulatorModel/Soft Robotic Manipulator Dynamic Model/Elastic Term ==
  data: k input; K output
function K = fcn(k)

K = [k(1) 0; 0 k(2)];

== matlab function SoftManipulatorModel/Soft Robotic Manipulator Dynamic Model/ Dissipative Term ==
  data: d input; D output
function D = fcn(d)

D = [d(1) 0; 0 d(2)];

== matlab function SoftManipulatorModel/Controller/Inertia Matrix ==
  data: q input; Dq output; m input; l input
function Dq = fcn(q,m,l)

q1 = q(1);
q2 = q(2);
m1 = m(1);
m2 = m(2);
l1 = l(1);
l2 = l(2);

Dq = zeros(2,2);
% fake_zero = 1e-3;
% tolerance = 1e-3;

% This equation got from Matlab symbolic calculation
% if abs(q1) < tolerance && abs(q2) > tolerance
%     Dq(1,1) = m2*((l1 + (l2*sin(q2))/(2*q2))*(conj(l1) + (sin(conj(q2))*conj(l2))/(2*conj(q2))) + (l2*conj(l2)*(cos(q2) - 1)*(cos(conj(q2)) - 1))/(4*q2*conj(q2))) + (l1*m1*conj(l1))/4;
%     Dq(1,2) = m2*((l2*sin(q2)*(conj(l1) + (sin(conj(q2))*conj(l2))/(2*conj(q2))))/(2*q2) + (l2*conj(l2)*(cos(q2) - 1)*(cos(conj(q2)) - 1))/(4*q2*conj(q2)));
%     Dq(2,1) = m2*((sin(conj(q2))*conj(l2)*(l1 + (l2*sin(q2))/(2*q2)))/(2*conj(q2)) + (l2*conj(l2)*(cos(q2) - 1)*(cos(conj(q2)) - 1))/(4*q2*conj(q2)));
%     Dq(2,2) = m2*((l2*conj(l2)*(cos(q2) - 1)*(cos(conj(q2)) - 1))/(4*q2*conj(q2)) + (l2*sin(conj(q2))*conj(l2)*sin(q2))/(4*q2*conj(q2)));
% elseif abs(q1) < tolerance && abs(q2) < tolerance
%     Dq(1,1) = (l1*m1*conj(l1))/4 + m2*(conj(l1) + conj(l2)/2)*(l1 + l2/2);
%     Dq(1,2) = (l2*m2*(conj(l1) + conj(l2)/2))/2;
%     Dq(2,1) = (m2*conj(l2)*(l1 + l2/2))/2;
%     Dq(2,2) = (l2*m2*conj(l2))/4;
% elseif abs(q1) > tolerance && abs(q2) < tolerance
%     Dq(1,1) = m1*((l1*conj(l1)*(cos(q1) - 1)*(cos(conj(q1)) - 1))/(4*q1*conj(q1)) + (l1*sin(conj(q1))*conj(l1)*sin(q1))/(4*q1*conj(q1))) + m2*(((sin(conj(q1))*conj(l2))/2 - (conj(l1)*(cos(conj(q1)) - 1))/conj(q1))*((l2*sin(q1))/2 - (l1*(cos(q1) - 1))/q1) + ((cos(conj(q1))*conj(l2))/2 + (sin(conj(q1))*conj(l1))/conj(q1))*((l2*cos(q1))/2 + (l1*sin(q1))/q1));
%     Dq(1,2) = m2*((l2*cos(q1)*((cos(conj(q1))*conj(l2))/2 + (sin(conj(q1))*conj(l1))/conj(q1)))/2 + (l2*sin(q1)*((sin(conj(q1))*conj(l2))/2 - (conj(l1)*(cos(conj(q1)) - 1))/conj(q1)))/2);
%     Dq(2,1) = m2*((sin(conj(q1))*conj(l2)*((l2*sin(q1))/2 - (l1*(cos(q1) - 1))/q1))/2 + (cos(conj(q1))*conj(l2)*((l2*cos(q1))/2 + (l1*sin(q1))/q1))/2);
%     Dq(2,2) = m2*((l2*cos(conj(q1))*conj(l2)*cos(q1))/4 + (l2*sin(conj(q1))*conj(l2)*sin(q1))/4);
% elseif abs(q1) > tolerance && abs(q2) > tolerance
%     Dq(1,1) = m2*(((conj(l1)*(cos(conj(q1)) - 1))/conj(q1) + (cos(conj(q1))*conj(l2)*(cos(conj(q2)) - 1))/(2*conj(q2)) - (sin(conj(q1))*sin(conj(q2))*conj(l2))/(2*conj(q2)))*((l1*(cos(q1) - 1))/q1 - (l2*sin(q1)*sin(q2))/(2*q2) + (l2*cos(q1)*(cos(q2) - 1))/(2*q2)) + ((l1*sin(q1))/q1 + (l2*cos(q1)*sin(q2))/(2*q2) + (l2*sin(q1)*(cos(q2) - 1))/(2*q2))*((sin(conj(q1))*conj(l1))/conj(q1) + (sin(conj(q1))*conj(l2)*(cos(conj(q2)) - 1))/(2*conj(q2)) + (cos(conj(q1))*sin(conj(q2))*conj(l2))/(2*conj(q2)))) + m1*((l1*conj(l1)*(cos(q1) - 1)*(cos(conj(q1)) - 1))/(4*q1*conj(q1)) + (l1*sin(conj(q1))*conj(l1)*sin(q1))/(4*q1*conj(q1)));
%     Dq(1,2) = m2*(((l2*cos(q1)*sin(q2))/(2*q2) + (l2*sin(q1)*(cos(q2) - 1))/(2*q2))*((sin(conj(q1))*conj(l1))/conj(q1) + (sin(conj(q1))*conj(l2)*(cos(conj(q2)) - 1))/(2*conj(q2)) + (cos(conj(q1))*sin(conj(q2))*conj(l2))/(2*conj(q2))) - ((l2*sin(q1)*sin(q2))/(2*q2) - (l2*cos(q1)*(cos(q2) - 1))/(2*q2))*((conj(l1)*(cos(conj(q1)) - 1))/conj(q1) + (cos(conj(q1))*conj(l2)*(cos(conj(q2)) - 1))/(2*conj(q2)) - (sin(conj(q1))*sin(conj(q2))*conj(l2))/(2*conj(q2))));
%     Dq(2,1) = m2*(((sin(conj(q1))*conj(l2)*(cos(conj(q2)) - 1))/(2*conj(q2)) + (cos(conj(q1))*sin(conj(q2))*conj(l2))/(2*conj(q2)))*((l1*sin(q1))/q1 + (l2*cos(q1)*sin(q2))/(2*q2) + (l2*sin(q1)*(cos(q2) - 1))/(2*q2)) + ((cos(conj(q1))*conj(l2)*(cos(conj(q2)) - 1))/(2*conj(q2)) - (sin(conj(q1))*sin(conj(q2))*conj(l2))/(2*conj(q2)))*((l1*(cos(q1) - 1))/q1 - (l2*sin(q1)*sin(q2))/(2*q2) + (l2*cos(q1)*(cos(q2) - 1))/(2*q2)));
%     Dq(2,2) = m2*(((l2*cos(q1)*sin(q2))/(2*q2) + (l2*sin(q1)*(cos(q2) - 1))/(2*q2))*((sin(conj(q1))*conj(l2)*(cos(conj(q2)) - 1))/(2*conj(q2)) + (cos(conj(q1))*sin(conj(q2))*conj(l2))/(2*conj(q2))) - ((l2*sin(q1)*sin(q2))/(2*q2) - (l2*cos(q1)*(cos(q2) - 1))/(2*q2))*((cos(conj(q1))*conj(l2)*(cos(conj(q2)) - 1))/(2*conj(q2)) - (sin(conj(q1))*sin(conj(q2))*conj(l2))/(2*conj(q2))));
% end

% if abs(q1) < tolerance && abs(q2) > tolerance
%     if q1 < 0
%         q1 = -fake_zero;
%     else
%         q1 = fake_zero;
%     end
% elseif abs(q1) < tolerance && abs(q2) < tolerance
%     if q1 < 0
%         q1 = -fake_zero;
%     else
%         q1 = fake_zero;
%     end
%     
%     if q2 < 0
%         q2 = -fake_zero;
%     else
%         q2 = fake_zero;
%     end
% elseif abs(q1) > tolerance && abs(q2) < tolerance
%     if q2 < 0
%         q2 = -fake_zero;
%     else
%         q2 = fake_zero;
%     end
% end

Dq(1,1) = m2*(((conj(l1)*(cos(conj(q1)) - 1))/conj(q1) + (cos(conj(q1))*conj(l2)*(cos(conj(q2)) - 1))/(2*conj(q2)) - (sin(conj(q1))*sin(conj(q2))*conj(l2))/(2*conj(q2)))*((l1*(cos(q1) - 1))/q1 - (l2*sin(q1)*sin(q2))/(2*q2) + (l2*cos(q1)*(cos(q2) - 1))/(2*q2)) + ((l1*sin(q1))/q1 + (l2*cos(q1)*sin(q2))/(2*q2) + (l2*sin(q1)*(cos(q2) - 1))/(2*q2))*((sin(conj(q1))*conj(l1))/conj(q1) + (sin(conj(q1))*conj(l2)*(cos(conj(q2)) - 1))/(2*conj(q2)) + (cos(conj(q1))*sin(conj(q2))*conj(l2))/(2*conj(q2)))) + m1*((l1*conj(l1)*(cos(q1) - 1)*(cos(conj(q1)) - 1))/(4*q1*conj(q1)) + (l1*sin(conj(q1))*conj(l1)*sin(q1))/(4*q1*conj(q1)));
Dq(1,2) = m2*(((l2*cos(q1)*sin(q2))/(2*q2) + (l2*sin(q1)*(cos(q2) - 1))/(2*q2))*((sin(conj(q1))*conj(l1))/conj(q1) + (sin(conj(q1))*conj(l2)*(cos(conj(q2)) - 1))/(2*conj(q2)) + (cos(conj(q1))*sin(conj(q2))*conj(l2))/(2*conj(q2))) - ((l2*sin(q1)*sin(q2))/(2*q2) - (l2*cos(q1)*(cos(q2) - 1))/(2*q2))*((conj(l1)*(cos(conj(q1)) - 1))/conj(q1) + (cos(conj(q1))*conj(l2)*(cos(conj(q2)) - 1))/(2*conj(q2)) - (sin(conj(q1))*sin(conj(q2))*conj(l2))/(2*conj(q2))));
Dq(2,1) = m2*(((sin(conj(q1))*conj(l2)*(cos(conj(q2)) - 1))/(2*conj(q2)) + (cos(conj(q1))*sin(conj(q2))*conj(l2))/(2*conj(q2)))*((l1*sin(q1))/q1 + (l2*cos(q1)*sin(q2))/(2*q2) + (l2*sin(q1)*(cos(q2) - 1))/(2*q2)) + ((cos(conj(q1))*conj(l2)*(cos(conj(q2)) - 1))/(2*conj(q2)) - (sin(conj(q1))*sin(conj(q2))*conj(l2))/(2*conj(q2)))*((l1*(cos(q1) - 1))/q1 - (l2*sin(q1)*sin(q2))/(2*q2) + (l2*cos(q1)*(cos(q2) - 1))/(2*q2)));
Dq(2,2) = m2*(((l2*cos(q1)*sin(q2))/(2*q2) + (l2*sin(q1)*(cos(q2) - 1))/(2*q2))*((sin(conj(q1))*conj(l2)*(cos(conj(q2)) - 1))/(2*conj(q2)) + (cos(conj(q1))*sin(conj(q2))*conj(l2))/(2*conj(q2))) - ((l2*sin(q1)*sin(q2))/(2*q2) - (l2*cos(q1)*(cos(q2) - 1))/(2*q2))*((cos(conj(q1))*conj(l2)*(cos(conj(q2)) - 1))/(2*conj(q2)) - (sin(conj(q1))*sin(conj(q2))*conj(l2))/(2*conj(q2))));

% for i = 1:2
%     for j = 1:2
%         if Dq(i,j) < tolerance
%             Dq(i,j) = 0;
%         end
%     end
% end
